simulink model "METI_Thermal_ver01_Jmaab_2018b"  (R2018b)
settings: Solver=ode8  StartTime=0  StopTime=end_time  FixedStep=sampling_time  RelTol=1e-3
PreLoadFcn:
  | %init_setting;
values from neighbouring files (symbols this model uses):
  degC2K = 273.15    [METI_TRAMI_Thermal_ver01_Jmaab_PreLoad.m]    (also in init_setting_METI.m)
  K2degC = -273.15    [METI_TRAMI_Thermal_ver01_Jmaab_PreLoad.m]    (also in init_setting_METI.m)
  sampling_time = 0.0025    [METI_TRAMI_Thermal_ver01_Jmaab_PreLoad.m]
undefined symbols (not defined in the file or in its folder): ACC_D_Gain, ACC_I_Gain, ACC_P_Gain, ALT_CNT_ALT_OFF_RPM_HYS_rpm, ALT_CNT_ALT_ON_RPM_HYS_rpm, ALT_CNT_Alter_V_BASE_V, ALT_CNT_Alter_V_Kaisei_V, ALT_CNT_flag_disable_kaisei, ALT_CNT_V_Battely_Kudo_V, ALT_PNT_ALT_GDCurrent_A, ALT_PNT_ALT_GDVolt_V, ALT_PNT_Alter_limit_Current_V_table, ALT_PNT_Alter_limit_Current_V_table_x_rpm, ALT_PNT_Alter_trq_Nm_map, ALT_PNT_Alter_trq_Nm_map_x_rpm, ALT_PNT_Alter_trq_Nm_map_y_Current_A, ALT_PNT_Alter_trq_Nm_map_z_Volt_tgt_V, ALT_PNT_eta_pulley_alt, ALT_PNT_Gain_Alt_v_del, ALT_PNT_ratio_pulley_alt, ALT_PNT_Tau_Alternator_V_tgt_s, ALT_PNT_trq_alter_output_LL_Nm, BK_PNT_Pow_UL, BK_PNT_Tau_brake, Brk_LL, Brk_PGain, Brk_UL, BT_PNT_Lo_Capa_lo_batt_F, BT_PNT_Lo_ocv_SOC_lo_batt_OCV_V_table, BT_PNT_Lo_ocv_SOC_lo_batt_OCV_V_table_x_SOC, BT_PNT_Lo_R_lo_batt_ohm, BT_PNT_Lo_SOC_MAX_lo_batt, BT_PNT_Lo_SOC_MIN_lo_batt, BT_PNT_Lo_SOC_START_lo_batt, BT_PNT_Lo_V_start_ocv, DF_PNT_DF_gear, DF_PNT_DFBlock2DFAir_Heat_Resi_KpW, DF_PNT_DFBlock_Heat_Capa_JpK, DF_PNT_DFBlock_Temp_ini_degC, DF_PNT_DFOil2DFBlock_Heat_Resi_KpW, DF_PNT_DFOil_Heat_Capa_JpK, DF_PNT_DFOil_Temp_ini_degC, DF_PNT_Driveshaft_damper, DF_PNT_Driveshaft_delta_radps_LL, DF_PNT_Driveshaft_delta_radps_UL, DF_PNT_Driveshaft_spring, DF_PNT_eta_DF, DF_PNT_Outtemp_degC, DF_PNT_TMBlock2DFBlock_Heat_Resi_KpW, Driver_Brake_Const1, Driver_Brake_Const3, Driver_Brake_Switch_Const2, Driver_Brk_sh, drivmode_ACC, drivmode_CONST, drivmode_GensokuKaisei, drivmode_GensokuRikko, drivmode_STOP, EL_PNT_R_bodyelec_lo_ohm, ENG_CNT_acc_idlestop ... (+137)
libraries: METI_Lib_vehicle_model x31, simulink x7, AZAPA_Lib_vehicle_model x1
(part 2 of 4)

== system METI_Thermal_ver01_Jmaab_2018b/Vehicle/CNT/ENG_CNT ==
  Driver_Input : Inport
  sensor_VL_PNT_BUS : Inport  Port=2
  sensor_ENG_PNT : Inport  Port=3
  Bus Creator : BusCreator  Inputs=4
  Bus Creator1 : BusCreator  Inputs=10
  Bus Selector1 : BusSelector  OutputSignals=flag_Lockup
  Bus Selector12 : BusSelector  OutputSignals=v_VL_PNT_kmph
  Bus Selector13 : BusSelector  OutputSignals=n_eng_rpm,fuel_consumption,T_ENGTH_PNT_Coolant_degC
  Bus Selector14 : BusSelector  OutputSignals=open_accel_per,open_brake_per
  ENG_Cntrl : Subsystem
  ENG_CNT_out : Outport
  tag scope: ENG_CNT_CAN_Tx=scoped
  wires:
  Bus Creator/1 -> [ENG_CNT_CAN_Tx]  "ENG_CNT_CAN_Tx"
  ENG_Cntrl/1(open_throttle_per) -> Bus Creator/1, Bus Creator1/1
  ENG_Cntrl/2(flag_IdleStop) -> Bus Creator/2, Bus Creator1/2
  ENG_Cntrl/3(flag_fuelcut) -> Bus Creator/3, Bus Creator1/3
  ENG_Cntrl/4(fuel_ratio) -> Bus Creator1/4
  ENG_Cntrl/5(timing_ignition) -> Bus Creator1/5
  ENG_Cntrl/6(n_eng_rpm) -> Bus Creator/4, Bus Creator1/6
  ENG_Cntrl/7(flag_ON_Starter) -> Bus Creator1/7
  Bus Creator1/1 -> ENG_CNT_out/1  "ENG_CNT_out"
  sensor_ENG_PNT/1 -> Bus Selector13/1
  Bus Selector13/1 -> ENG_Cntrl/3(sens_ENG_PNT)  "<n_eng_rpm>"
  sensor_VL_PNT_BUS/1 -> Bus Selector12/1
  Bus Selector12/1 -> ENG_Cntrl/6(v_VL_PNT_kmph)  "<v_VL_PNT_kmph>"
  Driver_Input/1 -> Bus Selector14/1
  Bus Selector14/1 -> ENG_Cntrl/1(open_accel_per)  "<open_accel_per>"
  Bus Selector14/2 -> ENG_Cntrl/2(open_brake_per)  "<open_brake_per>"
  [ENG_CNT_CAN_Rx] -> Bus Selector1/1
  Bus Selector1/1 -> ENG_Cntrl/7(flag_Lockup)  "<flag_Lockup>"
  ENG_Cntrl/8(K_Fuel) -> Bus Creator1/8
  ENG_Cntrl/9(V_ENG_CNT_WP_V) -> Bus Creator1/9
  ENG_Cntrl/10(V_ENG_CNT_RDFan_V) -> Bus Creator1/10
  Bus Selector13/2 -> ENG_Cntrl/4(fuel_consumption)  "<fuel_consumption>"
  Bus Selector13/3 -> ENG_Cntrl/5(T_ENGTH_PNT_Coolant_K)  "<T_ENGTH_PNT_Coolant_degC>"

== system METI_Thermal_ver01_Jmaab_2018b/Vehicle/CNT/TM_CNT ==
  sensor_VL_PNT_BUS : Inport
  sensor_ENG_PNT : Inport  Port=2
  sensor_TM_PNT_BUS : Inport  Port=3
  Bus Creator : BusCreator  Inputs=2
  Bus Creator1 : BusCreator  Inputs=4
  Bus Selector1 : BusSelector  OutputSignals=open_throttle_per
  Bus Selector2 : BusSelector  OutputSignals=n_TM_PNT_rpm,T_TMTH_PNT_CVTF_degC
  Bus Selector3 : BusSelector  OutputSignals=v_VL_PNT_kmph
  Bus Selector4 : BusSelector  OutputSignals=T_ENGTH_PNT_Coolant_degC
  TM_Ctrl : Subsystem
  TM_CNT_out : Outport
  tag scope: TM_CNT_CAN_Tx=scoped
  wires:
  Bus Creator/1 -> [TM_CNT_CAN_Tx]  "TM_CNT_CAN_Tx"
  [TM_CNT_CAN_Rx] -> Bus Selector1/1
  Bus Selector1/1 -> TM_Ctrl/5(open_throttle_per)  "<open_throttle_per>"
  TM_Ctrl/1(flag_Lockup) -> Bus Creator1/1, Bus Creator/1
  TM_Ctrl/2(omg_Slip_rpm) -> Bus Creator1/2, Bus Creator/2
  TM_Ctrl/3(ratio_CVT) -> Bus Creator1/3
  Bus Creator1/1 -> TM_CNT_out/1  "TM_CNT_out"
  sensor_VL_PNT_BUS/1 -> Bus Selector3/1
  Bus Selector3/1 -> TM_Ctrl/1(v_VL_PNT_kmph)  "<v_VL_PNT_kmph>"
  sensor_TM_PNT_BUS/1 -> Bus Selector2/1
  Bus Selector2/1 -> TM_Ctrl/2(n_TM_PNT_rpm)  "<n_TM_PNT_rpm>"
  TM_Ctrl/4(R_CVTF_warmer_tgt_KpW) -> Bus Creator1/4
  sensor_ENG_PNT/1 -> Bus Selector4/1
  Bus Selector2/2 -> TM_Ctrl/3(T_TMTH_PNT_CVTF_K)  "<T_TMTH_PNT_CVTF_degC>"
  Bus Selector4/1 -> TM_Ctrl/4(T_ENG_Coolant_K)  "<T_ENGTH_PNT_Coolant_degC>"

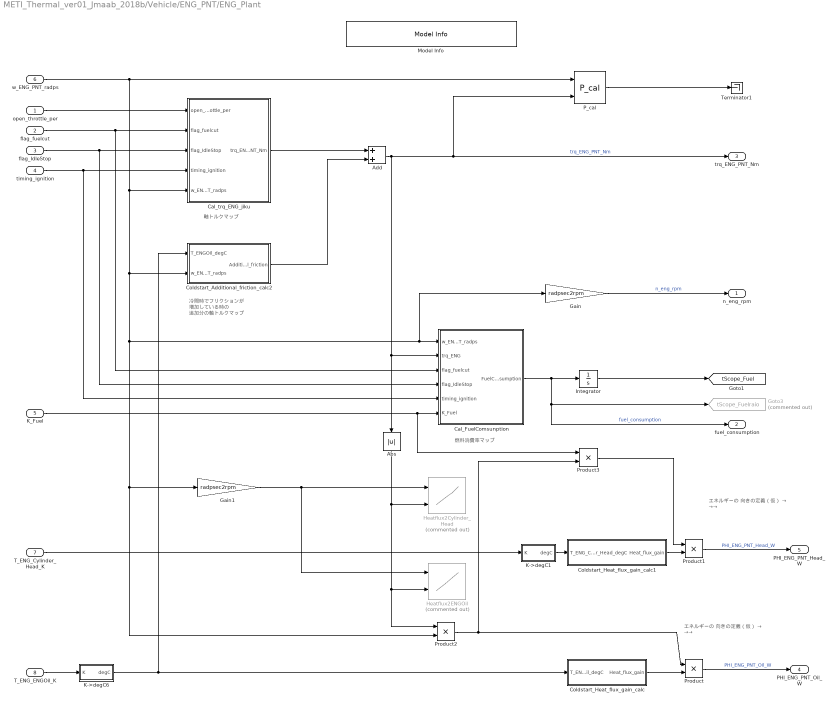
== system METI_Thermal_ver01_Jmaab_2018b/Vehicle/ENG_PNT/ENG_Plant ==
  note: 軸トルクマップ
  note: 燃料消費率マップ
  note: 冷間時でフリクションが
      | 増加している時の
      | 追加分の軸トルクマップ
  note: エネルギーの
      | 向きの定義（仮）
      | → →→
  note: エネルギーの
      | 向きの定義（仮）
      | → →→
  open_throttle_per : Inport
  flag_fuelcut : Inport  Port=2
  flag_IdleStop : Inport  Port=3
  timing_ignition : Inport  Port=4
  K_Fuel : Inport  Port=5
  w_ENG_PNT_radps : Inport  Port=6
  T_ENG_Cylinder_Head_K : Inport  Port=7
  T_ENG_ENGOil_K : Inport  Port=8
  Abs : Abs
  Add : Sum
  Cal_FuelComsunption : Subsystem
  Cal_trq_ENG_jiku : Subsystem
  Coldstart_Additional_friction_calc2 : Subsystem
  Coldstart_Heat_flux_gain_calc : Subsystem
  Coldstart_Heat_flux_gain_calc1 : Subsystem
  Gain : Gain  Gain=radpsec2rpm
  Gain1 : Gain  Gain=radpsec2rpm
  Goto3 : Goto  Commented=on  GotoTag=tScope_Fuelraio  TagVisibility=global
  Heatflux2Cylinder_Head : Lookup_n-D  Commented=on  BreakpointsForDimension1=ENG_PNT_Heatflux2Cylinder_Head_W_x_rpm  BreakpointsForDimension2=ENG_PNT_Heatflux2Cylinder_Head_W_y_trq  Table=ENG_PNT_Heatflux2Cylinder_Head_W  InternalRulePriority=Speed  RndMeth=Simplest  InputSameDT=on
  Heatflux2ENGOil : Lookup_n-D  Commented=on  BreakpointsForDimension1=ENG_PNT_Heatflux2ENGOil_W_x_rpm  BreakpointsForDimension2=ENG_PNT_Heatflux2ENGOil_W_y_trq  Table=ENG_PNT_Heatflux2ENGOil_W  InternalRulePriority=Speed  RndMeth=Simplest  InputSameDT=on
  Integrator : Integrator
  K->degC1 : Subsystem
  K->degC6 : Subsystem
  Model Info : simulink/Model-Wide Utilities/Model Info  Frame=on  DisplayStringWithTags=【注記】 ・エンジンモデルはトルク出力動作させる側が正  HorizontalTextAlignment=Left  LeftAlignmentValue=0.02
  P_cal : METI_Lib_vehicle_model/P_cal  Type_energy=回転運動  Type_output_energy=出力  Power_name=Po_  t_Workspace_Name=ENG_PNT_MECK  P_VariableName=Po_ENG_PNT_MECK  Across_VariableName=w_ENG_PNT_MECK  Throgh_VariableName=tq_ENG_PNT_MECK
  Product{,1..3} (4 alike) : Product
  Terminator1 : Terminator
  n_eng_rpm : Outport
  fuel_consumption : Outport  Port=2
  trq_ENG_PNT_Nm : Outport  Port=3
  PHI_ENG_PNT_Oil_W : Outport  Port=4
  PHI_ENG_PNT_Head_W : Outport  Port=5
  tag scope: tScope_Fuel=global
  wires:
  Cal_FuelComsunption/1(FuelConsumption) -> fuel_consumption/1, Goto3/1, Integrator/1  "fuel_consumption"
  Integrator/1 -> [tScope_Fuel]
  w_ENG_PNT_radps/1 -> P_cal/1, Coldstart_Additional_friction_calc2/2(w_ENG_PNT_radps), Gain1/1, Product2/2, Gain/1, Cal_FuelComsunption/1(w_ENG_PNT_radps), Cal_trq_ENG_jiku/5(w_ENG_PNT_radps)
  P_cal/1 -> Terminator1/1
  flag_fuelcut/1 -> Cal_trq_ENG_jiku/2(flag_fuelcut), Cal_FuelComsunption/3(flag_fuelcut)
  flag_IdleStop/1 -> Cal_FuelComsunption/4(flag_IdleStop), Cal_trq_ENG_jiku/3(flag_IdleStop)
  open_throttle_per/1 -> Cal_trq_ENG_jiku/1(open_throttle_per)
  Cal_trq_ENG_jiku/1(trq_ENG_PNT_Nm) -> Add/1
  timing_ignition/1 -> Cal_FuelComsunption/5(timing_ignition), Cal_trq_ENG_jiku/4(timing_ignition)
  Gain/1 -> n_eng_rpm/1  "n_eng_rpm"
  K->degC6/1(degC) -> Coldstart_Heat_flux_gain_calc/1(T_ENGOil_degC), Coldstart_Additional_friction_calc2/1(T_ENGOil_degC)
  T_ENG_Cylinder_Head_K/1 -> K->degC1/1(K)
  Product1/1 -> PHI_ENG_PNT_Head_W/1  "PHI_ENG_PNT_Head_W"
  Product/1 -> PHI_ENG_PNT_Oil_W/1  "PHI_ENG_PNT_Oil_W"
  Gain1/1 -> Heatflux2ENGOil/1, Heatflux2Cylinder_Head/1
  Coldstart_Heat_flux_gain_calc/1(Heat_flux_gain) -> Product/2
  Product2/1 -> Product/1, Product3/2
  Coldstart_Heat_flux_gain_calc1/1(Heat_flux_gain) -> Product1/2
  Coldstart_Additional_friction_calc2/1(Additional_friction) -> Add/2
  Add/1 -> trq_ENG_PNT_Nm/1, P_cal/2, Cal_FuelComsunption/2(trq_ENG), Abs/1  "trq_ENG_PNT_Nm"
  K_Fuel/1 -> Product3/1, Cal_FuelComsunption/6(K_Fuel)
  Abs/1 -> Product2/1, Heatflux2ENGOil/2, Heatflux2Cylinder_Head/2
  Product3/1 -> Product1/1
  T_ENG_ENGOil_K/1 -> K->degC6/1(K)
  K->degC1/1(degC) -> Coldstart_Heat_flux_gain_calc1/1(T_ENG_Cylinder_Head_degC)

== system METI_Thermal_ver01_Jmaab_2018b/Vehicle/ENG_PNT/K->degC ==
  K : Inport
  Constant2 : Constant  Value=K2degC
  Sum : Sum  Inputs=++|
  degC : Outport
  wires:
  K/1 -> Sum/2
  Constant2/1 -> Sum/1
  Sum/1 -> degC/1

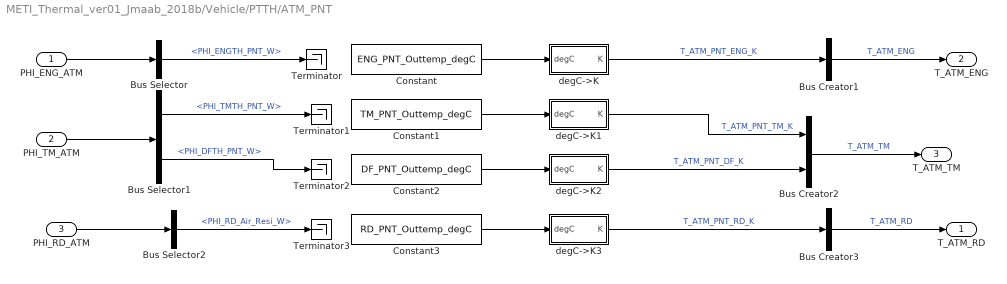
== system METI_Thermal_ver01_Jmaab_2018b/Vehicle/PTTH/ATM_PNT ==
  PHI_ENG_ATM : Inport
  PHI_TM_ATM : Inport  Port=2
  PHI_RD_ATM : Inport  Port=3
  Bus Creator1 : BusCreator  Inputs=1
  Bus Creator2 : BusCreator  Inputs=2
  Bus Creator3 : BusCreator  Inputs=1
  Bus Selector : BusSelector  OutputSignals=PHI_ENGTH_PNT_W
  Bus Selector1 : BusSelector  OutputSignals=PHI_TMTH_PNT_W,PHI_DFTH_PNT_W
  Bus Selector2 : BusSelector  OutputSignals=PHI_RD_Air_Resi_W
  Constant : Constant  Value=ENG_PNT_Outtemp_degC
  Constant1 : Constant  Value=TM_PNT_Outtemp_degC
  Constant2 : Constant  Value=DF_PNT_Outtemp_degC
  Constant3 : Constant  Value=RD_PNT_Outtemp_degC
  Terminator{,1..3} (4 alike) : Terminator
  degC->K : Subsystem
  degC->K1 : Subsystem
  degC->K2 : Subsystem
  degC->K3 : Subsystem
  T_ATM_RD : Outport
  T_ATM_ENG : Outport  Port=2
  T_ATM_TM : Outport  Port=3
  wires:
  Constant/1 -> degC->K/1(degC)
  Constant1/1 -> degC->K1/1(degC)
  Constant2/1 -> degC->K2/1(degC)
  Constant3/1 -> degC->K3/1(degC)
  Bus Selector1/2 -> Terminator2/1  "<PHI_DFTH_PNT_W>"
  degC->K/1(K) -> Bus Creator1/1  "T_ATM_PNT_ENG_K"
  degC->K1/1(K) -> Bus Creator2/1  "T_ATM_PNT_TM_K"
  degC->K2/1(K) -> Bus Creator2/2  "T_ATM_PNT_DF_K"
  degC->K3/1(K) -> Bus Creator3/1  "T_ATM_PNT_RD_K"
  PHI_ENG_ATM/1 -> Bus Selector/1
  Bus Selector/1 -> Terminator/1  "<PHI_ENGTH_PNT_W>"
  PHI_TM_ATM/1 -> Bus Selector1/1
  Bus Selector1/1 -> Terminator1/1  "<PHI_TMTH_PNT_W>"
  Bus Creator2/1 -> T_ATM_TM/1  "T_ATM_TM"
  Bus Creator1/1 -> T_ATM_ENG/1  "T_ATM_ENG"
  Bus Creator3/1 -> T_ATM_RD/1  "T_ATM_RD"
  PHI_RD_ATM/1 -> Bus Selector2/1
  Bus Selector2/1 -> Terminator3/1  "<PHI_RD_Air_Resi_W>"

== system METI_Thermal_ver01_Jmaab_2018b/Vehicle/PTTH/DTTH_PNT ==
  note: DFブロックへ
      | 放熱する熱量
  note: CVTFからエンジン冷却水へ
      | 放熱する熱量
  note: エンジンブロックからT/Mブロックへ
      | 放熱する熱量
  note: エネルギーの
      | 向きの定義（仮）
      | →→→
  note: エネルギーの
      | 向きの定義（仮）
      | →→→
  note: エネルギーの
      | 向きの定義（仮）
      | →→→
  note: T/MからCVTFへ
      | 放熱する熱量
  note: DFの損失が
      | DFオイルへの熱量
  TM_CNT_out : Inport
  T_ATM_TM : Inport  Port=2
  T_ENG_TM : Inport  Port=3
  PHI_TM_PNT_BUS : Inport  Port=4
  Bus Creator{1..4} (4 alike) : BusCreator  Inputs=2
  Bus Selector1 : BusSelector  OutputSignals=T_ENG_Block_K,T_ENGTH_PNT_Coolant_K
  Bus Selector2 : BusSelector  OutputSignals=R_CVTF_warmer_tgt_KpW
  Bus Selector3 : BusSelector  OutputSignals=Q_Tire_rol_resi,W_TM_PNT_W
  Bus Selector4 : BusSelector  OutputSignals=T_ATM_PNT_TM_K,T_ATM_PNT_DF_K
  DFTH_PNT : Subsystem
      mask Display: image(imread('picture\differential.png'))
  TMTH_PNT : Subsystem
      mask Display: image(imread('picture\image\transmission02.jpg'))
  Terminator : Terminator
  T_TMTH_PNT : Outport
  PHI_TM_ATM : Outport  Port=2
  PHI_TM_ENG : Outport  Port=3
  TMTH_Info : Outport  Port=4
  wires:
  DFTH_PNT/2(PHI_DFTH_PNT_W) -> Bus Creator3/1
  Bus Selector4/2 -> DFTH_PNT/3(T_ATM_PNT_DF_K)  "<T_ATM_PNT_DF_K>"
  TMTH_PNT/4(T_TMTH_PNT_CVTF_K) -> Terminator/1
  TMTH_PNT/2(T_TM_Block0_K) -> DFTH_PNT/1(T_DF_Block_K)
  DFTH_PNT/1(PHI_DF_Block_W) -> TMTH_PNT/1(W_TM_Block0_W)
  TMTH_PNT/6(PHI_TMTH_PNT_W) -> Bus Creator3/2
  TMTH_PNT/5(PHI_ENGBlock_Resi2_W) -> Bus Creator1/2
  TMTH_PNT/3(PHI_TM_CVTF_Resi_W) -> Bus Creator1/1
  T_ENG_TM/1 -> Bus Selector1/1
  Bus Selector1/1 -> TMTH_PNT/4(T_TM_Block_Resi_K)  "<T_ENG_Block_K>"
  Bus Selector1/2 -> TMTH_PNT/5(T_ENGTH_PNT_Coolant_K)  "<T_ENGTH_PNT_Coolant_K>"
  TMTH_PNT/1(T_TMTH_PNT_CVTF1_K) -> Bus Creator4/1, Bus Creator2/1  "T_TMTH_PNT_CVTF_K"
  DFTH_PNT/3(T_DFBlock_K) -> Bus Creator4/2, Bus Creator2/2  "T_DFBlock_K"
  Bus Creator2/1 -> T_TMTH_PNT/1  "T_TMTH_PNT"
  Bus Creator1/1 -> PHI_TM_ENG/1  "PHI_TM_ENG"
  Bus Creator3/1 -> PHI_TM_ATM/1  "PHI_TM_ATM"
  Bus Creator4/1 -> TMTH_Info/1  "TMTH_Info"
  PHI_TM_PNT_BUS/1 -> Bus Selector3/1
  Bus Selector3/2 -> TMTH_PNT/3(PHI_TM_PNT_W)  "<W_TM_PNT_W>"
  Bus Selector3/1 -> DFTH_PNT/2(PHI_DF_PNT_W)  "<Q_Tire_rol_resi>"
  TM_CNT_out/1 -> Bus Selector2/1
  Bus Selector2/1 -> TMTH_PNT/2(R_CVTF_warmer_tgt_KpW)  "<R_CVTF_warmer_tgt_KpW>"
  T_ATM_TM/1 -> Bus Selector4/1
  Bus Selector4/1 -> TMTH_PNT/6(T_ATM_PNT_TM_K)  "<T_ATM_PNT_TM_K>"

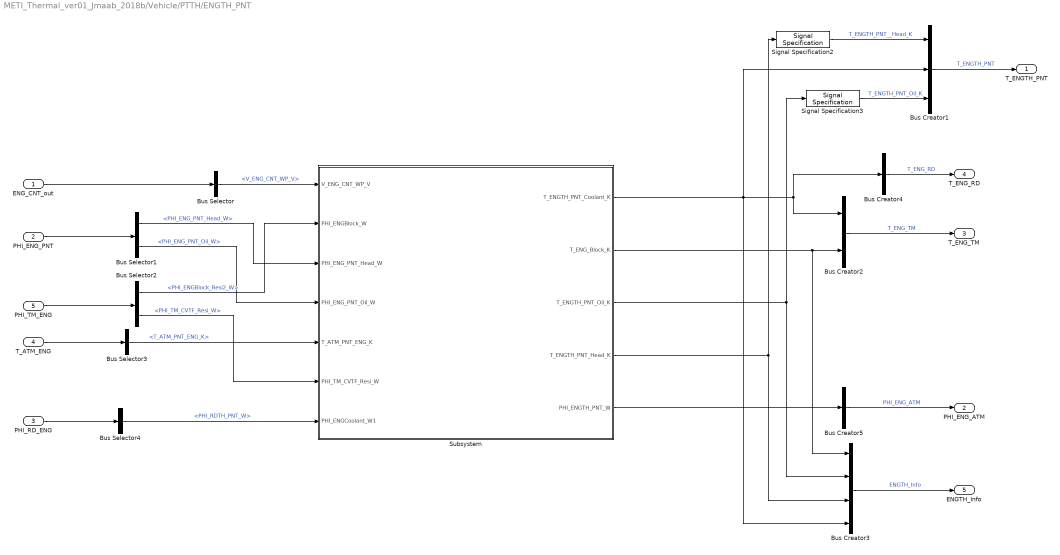
== system METI_Thermal_ver01_Jmaab_2018b/Vehicle/PTTH/ENGTH_PNT ==
  ENG_CNT_out : Inport
  PHI_ENG_PNT : Inport  Port=2
  PHI_RD_ENG : Inport  Port=3
  T_ATM_ENG : Inport  Port=4
  PHI_TM_ENG : Inport  Port=5
  Bus Creator1 : BusCreator  Inputs=3
  Bus Creator2 : BusCreator  Inputs=2
  Bus Creator3 : BusCreator  Inputs=4
  Bus Creator4 : BusCreator  Inputs=1
  Bus Creator5 : BusCreator  Inputs=1
  Bus Selector : BusSelector  OutputSignals=V_ENG_CNT_WP_V
  Bus Selector1 : BusSelector  OutputSignals=PHI_ENG_PNT_Head_W,PHI_ENG_PNT_Oil_W
  Bus Selector2 : BusSelector  OutputSignals=PHI_ENGBlock_Resi2_W,PHI_TM_CVTF_Resi_W
  Bus Selector3 : BusSelector  OutputSignals=T_ATM_PNT_ENG_K
  Bus Selector4 : BusSelector  OutputSignals=PHI_RDTH_PNT_W
  Signal Specification2 : SignalSpecification
  Signal Specification3 : SignalSpecification
  Subsystem : Subsystem
  T_ENGTH_PNT : Outport
  PHI_ENG_ATM : Outport  Port=2
  T_ENG_TM : Outport  Port=3
  T_ENG_RD : Outport  Port=4
  ENGTH_Info : Outport  Port=5
  wires:
  ENG_CNT_out/1 -> Bus Selector/1
  Subsystem/1(T_ENGTH_PNT_Coolant_K) -> Bus Creator3/4, Bus Creator1/2, Bus Creator2/1, Bus Creator4/1
  Subsystem/2(T_ENG_Block_K) -> Bus Creator3/1, Bus Creator2/2
  Subsystem/3(T_ENGTH_PNT_Oil_K) -> Bus Creator3/2, Signal Specification3/1
  Subsystem/4(T_ENGTH_PNT_Head_K) -> Bus Creator3/3, Signal Specification2/1
  Subsystem/5(PHI_ENGTH_PNT_W) -> Bus Creator5/1
  Bus Selector/1 -> Subsystem/1(V_ENG_CNT_WP_V)  "<V_ENG_CNT_WP_V>"
  PHI_ENG_PNT/1 -> Bus Selector1/1
  Bus Selector1/1 -> Subsystem/3(PHI_ENG_PNT_Head_W)  "<PHI_ENG_PNT_Head_W>"
  Bus Selector1/2 -> Subsystem/4(PHI_ENG_PNT_Oil_W)  "<PHI_ENG_PNT_Oil_W>"
  Bus Creator1/1 -> T_ENGTH_PNT/1  "T_ENGTH_PNT"
  Signal Specification2/1 -> Bus Creator1/1  "T_ENGTH_PNT__Head_K"
  Signal Specification3/1 -> Bus Creator1/3  "T_ENGTH_PNT_Oil_K"
  Bus Creator2/1 -> T_ENG_TM/1  "T_ENG_TM"
  Bus Creator4/1 -> T_ENG_RD/1  "T_ENG_RD"
  Bus Creator5/1 -> PHI_ENG_ATM/1  "PHI_ENG_ATM"
  Bus Creator3/1 -> ENGTH_Info/1  "ENGTH_Info"
  PHI_TM_ENG/1 -> Bus Selector2/1
  Bus Selector2/1 -> Subsystem/2(PHI_ENGBlock_W)  "<PHI_ENGBlock_Resi2_W>"
  Bus Selector2/2 -> Subsystem/6(PHI_TM_CVTF_Resi_W)  "<PHI_TM_CVTF_Resi_W>"
  T_ATM_ENG/1 -> Bus Selector3/1
  PHI_RD_ENG/1 -> Bus Selector4/1
  Bus Selector3/1 -> Subsystem/5(T_ATM_PNT_ENG_K)  "<T_ATM_PNT_ENG_K>"
  Bus Selector4/1 -> Subsystem/7(PHI_ENGCoolant_W1)  "<PHI_RDTH_PNT_W>"

== system METI_Thermal_ver01_Jmaab_2018b/Vehicle/PTTH/RDTH_PNT ==
  ENG_CNT_out : Inport
  T_ENG_RD : Inport  Port=2
  v_VL_PNT_kmph : Inport  Port=3
  T_ATM_RD : Inport  Port=4
  Bus Creator1 : BusCreator  Inputs=1
  Bus Creator2 : BusCreator  Inputs=1
  Bus Creator4 : BusCreator  Inputs=2
  Bus Selector : BusSelector  OutputSignals=V_ENG_CNT_RDFan_V
  Bus Selector1 : BusSelector  OutputSignals=T_ENGTH_PNT_Coolant_K
  Bus Selector2 : BusSelector  OutputSignals=T_ATM_PNT_RD_K
  Subsystem : Subsystem
  mps2kmph : Gain  Gain=mps2kmph
  PHI_RD_ENG : Outport
  PHI_RD_ATM : Outport  Port=2
  RDTH_Info : Outport  Port=3
  wires:
  v_VL_PNT_kmph/1 -> mps2kmph/1
  Subsystem/1(T_RDCoolant_degC) -> Bus Creator4/1
  Subsystem/2(PHI_RDTH_PNT_W) -> Bus Creator4/2, Bus Creator1/1
  Subsystem/3(PHI_RD_Air_Resi_W) -> Bus Creator2/1
  ENG_CNT_out/1 -> Bus Selector/1
  Bus Selector/1 -> Subsystem/1(RD_PNT_Voltage_RDFan_V)  "<V_ENG_CNT_RDFan_V>"
  T_ENG_RD/1 -> Bus Selector1/1
  Bus Selector1/1 -> Subsystem/3(T_ENGTH_PNT_Coolant_K)  "<T_ENGTH_PNT_Coolant_K>"
  mps2kmph/1 -> Subsystem/2(v_VL_PNT_kmph)  "v_VL_PNT_kmph"
  Bus Creator4/1 -> RDTH_Info/1  "RDTH_Info"
  Bus Creator1/1 -> PHI_RD_ENG/1  "PHI_RD_ENG"
  Bus Creator2/1 -> PHI_RD_ATM/1  "PHI_RD_ATM"
  T_ATM_RD/1 -> Bus Selector2/1
  Bus Selector2/1 -> Subsystem/4(T_ATM_PNT_RD_K)  "<T_ATM_PNT_RD_K>"

== system METI_Thermal_ver01_Jmaab_2018b/Vehicle/TM_PNT/DF_PNT ==
  note: DF効率
  note: 車両を動かす側が正
  w_DF_PNT_DN_radps : Inport
  w_DF_PNT_UP_radps : Inport  Port=2
  T_DF_PNT_K : Inport  Port=3
  Constant4 : Constant  Value=DF_PNT_DF_gear
  DriveShaft : Subsystem
  Product4 : Product  Inputs=*/  RndMeth=Zero
  Product7 : Product  Inputs=*/  RndMeth=Zero
  Q_cal1 : METI_Lib_vehicle_model/P_cal  Type_energy=回転運動  Type_output_energy=出力  Power_name=Po_  t_Workspace_Name=DF_PNT_MECK  P_VariableName=Po_DF_PNT_MECK  Across_VariableName=w_DF_PNT_MECK  Throgh_VariableName=tq_DF_PNT_MECK
  Q_cal4 : METI_Lib_vehicle_model/P_cal  Type_energy=回転運動  Type_output_energy=損失  Power_name=Pl_  t_Workspace_Name=DF_PNT_MECK_LOSS  P_VariableName=Pl_DF_PNT_MECK_LOSS  Across_VariableName=w_DF_PNT_MECK_LOSS  Throgh_VariableName=tq_DF_PNT_MECK_LOSS
  Terminator : Terminator
  Terminator3 : Terminator
  eta_DF : Constant  Value=DF_PNT_eta_DF
  eta_cal : METI_Lib_vehicle_model/eta_cal  SystemSampleTime=-1
  trq_DS_PNT_Nm : Outport
  trq_DFNT_Nm : Outport  Port=2
  PHI_DF_PNT_W : Outport  Port=3
  wires:
  w_DF_PNT_UP_radps/1 -> Product4/1, Q_cal4/1, Q_cal1/1
  eta_DF/1 -> eta_cal/1
  eta_cal/2 -> Q_cal1/2, trq_DFNT_Nm/1  "trq_DFNT_Nm"
  eta_cal/1 -> Q_cal4/2
  Q_cal1/1 -> Terminator3/1
  Constant4/1 -> Product7/2, Product4/2
  Product7/1 -> eta_cal/2
  DriveShaft/1(trq_DS_PNT_in_Nm) -> trq_DS_PNT_Nm/1  "trq_DS_PNT_Nm"
  Product4/1 -> DriveShaft/2(w_DS_PNT_in_radps)
  w_DF_PNT_DN_radps/1 -> DriveShaft/1(w_TR_PNT_radps)
  DriveShaft/2(trq_DF_PNT_Nm) -> Product7/1
  Q_cal4/1 -> PHI_DF_PNT_W/1
  T_DF_PNT_K/1 -> Terminator/1

== system METI_Thermal_ver01_Jmaab_2018b/Vehicle/TM_PNT/K->degC ==
  K : Inport
  Constant2 : Constant  Value=K2degC
  Sum : Sum  Inputs=++|
  degC : Outport
  wires:
  K/1 -> Sum/2
  Constant2/1 -> Sum/1
  Sum/1 -> degC/1

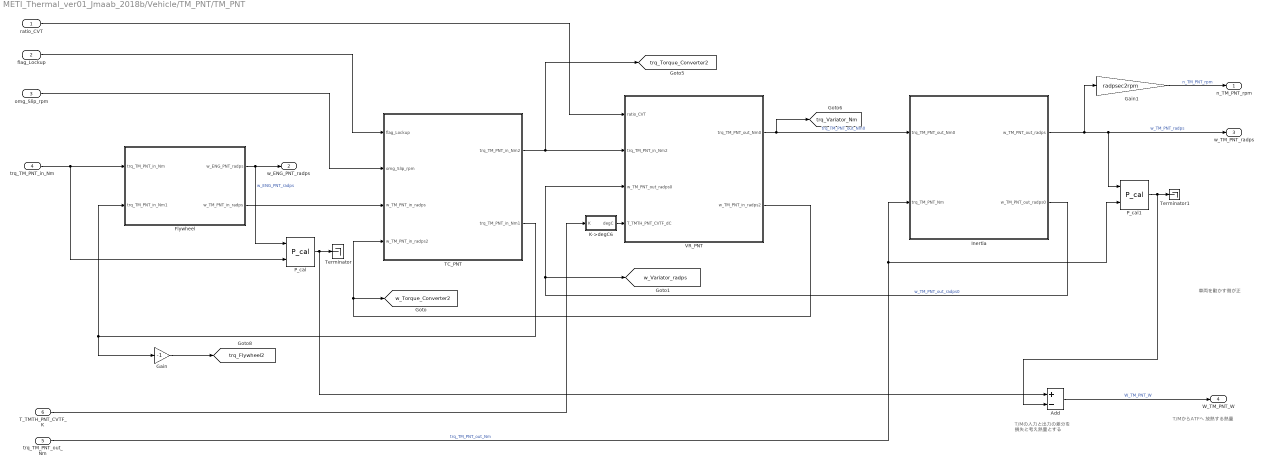
== system METI_Thermal_ver01_Jmaab_2018b/Vehicle/TM_PNT/TM_PNT ==
  note: 車両を動かす側が正
  note: T/MからATFへ
      | 放熱する熱量
  note: T/Mの入力と出力の差分を
      | 損失と考え熱量とする
  ratio_CVT : Inport
  flag_Lockup : Inport  Port=2
  omg_Slip_rpm : Inport  Port=3
  trq_TM_PNT_in_Nm : Inport  Port=4
  trq_TM_PNT_out_Nm : Inport  Port=5
  T_TMTH_PNT_CVTF_K : Inport  Port=6
  Add : Sum  Inputs=+-
  Flywheel : Subsystem
  Gain : Gain  Gain=-1
  Gain1 : Gain  Gain=radpsec2rpm
  Inertia : Subsystem
  K->degC6 : Subsystem
  P_cal : METI_Lib_vehicle_model/P_cal  Type_energy=回転運動  Type_output_energy=出力  Power_name=Po_  t_Workspace_Name=TM_PNT_MECK_UP  P_VariableName=Po_TM_PNT_MECK_UP  Across_VariableName=w_TM_PNT_MECK_UP  Throgh_VariableName=tq_TM_PNT_MECK_UP
  P_cal1 : METI_Lib_vehicle_model/P_cal  Type_energy=回転運動  Type_output_energy=出力  Power_name=Po_  t_Workspace_Name=TM_PNT_MECK_DN  P_VariableName=Po_TM_PNT_MECK_DN  Across_VariableName=w_TM_PNT_MECK_DN  Throgh_VariableName=tq_TM_PNT_MECK_DN
  TC_PNT : Subsystem
  Terminator : Terminator
  Terminator1 : Terminator
  VR_PNT : Subsystem
  n_TM_PNT_rpm : Outport
  w_ENG_PNT_radps : Outport  Port=2
  w_TM_PNT_radps : Outport  Port=3
  W_TM_PNT_W : Outport  Port=4
  tag scope: trq_Flywheel2=global, trq_Torque_Converter2=global, trq_Variator_Nm=global, w_Torque_Converter2=global, w_Variator_radps=global
  wires:
  VR_PNT/2(w_TM_PNT_in_radps2) -> [w_Torque_Converter2], TC_PNT/4(w_TM_PNT_in_radps2)
  TC_PNT/1(trq_TM_PNT_in_Nm2) -> [trq_Torque_Converter2], VR_PNT/2(trq_TM_PNT_in_Nm2)
  flag_Lockup/1 -> TC_PNT/1(flag_Lockup)
  omg_Slip_rpm/1 -> TC_PNT/2(omg_Slip_rpm)
  ratio_CVT/1 -> VR_PNT/1(ratio_CVT)
  TC_PNT/2(trq_TM_PNT_in_Nm1) -> Gain/1, Flywheel/2(trq_TM_PNT_in_Nm1)
  Flywheel/2(w_TM_PNT_in_radps) -> TC_PNT/3(w_TM_PNT_in_radps)
  Flywheel/1(w_ENG_PNT_radps) -> w_ENG_PNT_radps/1, P_cal/1  "w_ENG_PNT_radps"
  trq_TM_PNT_in_Nm/1 -> P_cal/2, Flywheel/1(trq_TM_PNT_in_Nm)
  Inertia/1(w_TM_PNT_out_radps) -> w_TM_PNT_radps/1, P_cal1/1, Gain1/1  "w_TM_PNT_radps"
  Gain1/1 -> n_TM_PNT_rpm/1  "n_TM_PNT_rpm"
  P_cal/1 -> Add/1, Terminator/1
  P_cal1/1 -> Terminator1/1, Add/2
  trq_TM_PNT_out_Nm/1 -> Inertia/2(trq_TM_PNT_Nm), P_cal1/2  "trq_TM_PNT_out_Nm"
  Inertia/2(w_TM_PNT_out_radps0) -> [w_Variator_radps], VR_PNT/3(w_TM_PNT_out_radps0)  "w_TM_PNT_out_radps0"
  VR_PNT/1(trq_TM_PNT_out_Nm0) -> [trq_Variator_Nm], Inertia/1(trq_TM_PNT_out_Nm0)  "trq_TM_PNT_out_Nm0"
  Add/1 -> W_TM_PNT_W/1  "W_TM_PNT_W"
  T_TMTH_PNT_CVTF_K/1 -> K->degC6/1(K)
  Gain/1 -> [trq_Flywheel2]
  K->degC6/1(degC) -> VR_PNT/4(T_TMTH_PNT_CVTF_dC)

== system METI_Thermal_ver01_Jmaab_2018b/Driver/Caliculate_Opeining_Accel/FB/Filter ==
  In1 : Inport
  Gain3 : Gain  Gain=10
  Gain4 : Gain  Gain=0.1
  Rounding Function : Rounding  Operator=round
  Out1 : Outport
  wires:
  Rounding Function/1 -> Gain4/1
  In1/1 -> Gain3/1
  Gain3/1 -> Rounding Function/1
  Gain4/1 -> Out1/1

== system METI_Thermal_ver01_Jmaab_2018b/Driver/Caliculate_Opeining_Accel/FF/Air_Resistance ==
  V_tgt : Inport
  V_wind : Constant  Value=VL_PNT_V_wind
  cal_Air_resi1 : METI_Lib_vehicle_model/vehicle_model/cal_Air_resi  Vel_max=200
  F_air_resi : Outport
  wires:
  V_tgt/1 -> cal_Air_resi1/1
  V_wind/1 -> cal_Air_resi1/2
  cal_Air_resi1/1 -> F_air_resi/1

== system METI_Thermal_ver01_Jmaab_2018b/Driver/Caliculate_Opeining_Accel/FF/Cal_M_ENG_jiku2 ==
  note: 軸トルクマップ
  FF_trq_accel_Nm : Inport
  pre_n_eng_rpm : Inport  Port=2
  2-D Lookup Table : Lookup_n-D  BreakpointsForDimension1=ENG_trq_rev  BreakpointsForDimension2=ENG_rpm  Table=ENG_throttle_rev  ExtrapMethod=Clip  UseLastTableValue=on  RndMeth=Simplest  InputSameDT=on
  2-D Lookup Table1 : Lookup_n-D  BreakpointsForDimension1=ENG_PNT_trq_Nm_map_y_throttle  BreakpointsForDimension2=ENG_PNT_trq_Nm_map_x_rpm  Table=ENG_PNT_trq_Nm_map  ExtrapMethod=Clip  UseLastTableValue=on  RndMeth=Simplest  InputSameDT=on
  Constant : Constant  Value=0
  Subsystem : Subsystem
  Sum : Sum  Inputs=|++
  FF_open_accel_per : Outport
  wires:
  FF_trq_accel_Nm/1 -> Sum/1
  2-D Lookup Table/1 -> Subsystem/1(In1)
  pre_n_eng_rpm/1 -> 2-D Lookup Table/2, 2-D Lookup Table1/2
  Constant/1 -> 2-D Lookup Table1/1
  Sum/1 -> 2-D Lookup Table/1
  2-D Lookup Table1/1 -> Sum/2
  Subsystem/1(Out1) -> FF_open_accel_per/1

== system METI_Thermal_ver01_Jmaab_2018b/Driver/Caliculate_Opeining_Accel/FF/Inertial_Resistance ==
  V_tgt : Inport
  Constant : Constant  Value=M
  Derivative : Derivative
  Divide : Product  OutDataTypeStr=Inherit: Same as first input
  F_Inertia : Outport
  wires:
  Constant/1 -> Divide/2
  Derivative/1 -> Divide/1
  Divide/1 -> F_Inertia/1
  V_tgt/1 -> Derivative/1

== system METI_Thermal_ver01_Jmaab_2018b/Driver/Caliculate_Opeining_Accel/FF/Rolling_Resistance ==
  note: 20151211修正
      |
      | 空気抵抗と表現を統一する、ため
      | -1のGainを削除
  V_tgt : Inport
  cal_roll_resi1 : METI_Lib_vehicle_model/vehicle_model/cal_roll_resi  Myu_tire=myu  Vehicle_Mass=M  Gravi_acc=g
  F_rollresi : Outport
  wires:
  V_tgt/1 -> cal_roll_resi1/1
  cal_roll_resi1/1 -> F_rollresi/1

== system METI_Thermal_ver01_Jmaab_2018b/Vehicle/ALT_PNT/Subsystem/I_alt_cal ==
  target_volt_ALT_V : Inport
  volt_BT_PNT_Lo_V : Inport  Port=2
  rpm_alt : Inport  Port=3
  Add : Sum
  Cal_I_alt_P_control : Subsystem
  Cal_I_alt_base : Subsystem
  Constant : Constant  Value=12
  Constant4 : Constant  Value=0
  Limit_Current_Max : Lookup_n-D  NumberOfTableDimensions=1  BreakpointsForDimension1=ALT_PNT_Alter_limit_Current_V_table_x_rpm  Table=ALT_PNT_Alter_limit_Current_V_table  ExtrapMethod=Clip  UseLastTableValue=on  RndMeth=Simplest  InputSameDT=on
  MinMax2 : MinMax  Function=max  Inputs=2
  Sum1 : Sum  Inputs=|+-
  Sum2 : Sum  Inputs=-+|
  電圧比較 : MinMax  Inputs=2
  I_alt : Outport
  wires:
  target_volt_ALT_V/1 -> Sum1/1, Sum2/2
  volt_BT_PNT_Lo_V/1 -> Sum2/1
  rpm_alt/1 -> Limit_Current_Max/1
  Constant4/1 -> MinMax2/2
  Limit_Current_Max/1 -> MinMax2/1  "I_limit_ALT"
  電圧比較/1 -> I_alt/1
  Add/1 -> 電圧比較/2
  Sum2/1 -> Cal_I_alt_P_control/1(V_delt_tgt)
  MinMax2/1 -> 電圧比較/1
  Constant/1 -> Sum1/2
  Sum1/1 -> Cal_I_alt_base/1(V_delt_tgt)
  Cal_I_alt_P_control/1(I_alt_base) -> Add/1
  Cal_I_alt_base/1(I_alt_base) -> Add/2

== system METI_Thermal_ver01_Jmaab_2018b/Vehicle/ALT_PNT/Subsystem/Torque_Guard ==
  current_ALT_PNT_A : Inport
  V_ALT_PNT : Inport  Port=2
  n_ROT_slavepulley12_rpm : Inport  Port=3
  ALT_GDCurrent : Inport  Port=4
  ALT_GDVolt : Inport  Port=5
  Caliculate_Axes_Torque1 : Lookup_n-D  NumberOfTableDimensions=3  BreakpointsForDimension1=ALT_PNT_Alter_trq_Nm_map_x_rpm  BreakpointsForDimension2=ALT_PNT_Alter_trq_Nm_map_y_Current_A  BreakpointsForDimension3=ALT_PNT_Alter_trq_Nm_map_z_Volt_tgt_V  Table=ALT_PNT_Alter_trq_Nm_map  RndMeth=Simplest  InputSameDT=on
  Caliculate_Axes_Torque2 : Lookup_n-D  NumberOfTableDimensions=3  BreakpointsForDimension1=ALT_PNT_Alter_trq_Nm_map_x_rpm  BreakpointsForDimension2=ALT_PNT_Alter_trq_Nm_map_y_Current_A  BreakpointsForDimension3=ALT_PNT_Alter_trq_Nm_map_z_Volt_tgt_V  Table=ALT_PNT_Alter_trq_Nm_map  RndMeth=Simplest  InputSameDT=on
  Constant3 : Constant  Value=ALT_PNT_trq_alter_output_LL_Nm
  MinMax : MinMax  Inputs=2
  MinMax1 : MinMax  Function=max  Inputs=2
  trq_trqsource : Outport
  wires:
  ALT_GDCurrent/1 -> Caliculate_Axes_Torque2/2
  Caliculate_Axes_Torque2/1 -> MinMax/2
  MinMax/1 -> MinMax1/1
  Caliculate_Axes_Torque1/1 -> MinMax/1
  Constant3/1 -> MinMax1/2
  ALT_GDVolt/1 -> Caliculate_Axes_Torque2/3
  MinMax1/1 -> trq_trqsource/1
  V_ALT_PNT/1 -> Caliculate_Axes_Torque1/3
  current_ALT_PNT_A/1 -> Caliculate_Axes_Torque1/2
  n_ROT_slavepulley12_rpm/1 -> Caliculate_Axes_Torque2/1, Caliculate_Axes_Torque1/1

== system METI_Thermal_ver01_Jmaab_2018b/Vehicle/BT_PNT_Lo/Cal_SOC/Subsystem4 ==
  In1 : Inport
  In2 : Inport  Port=2
  To Workspace : ToWorkspace  VariableName=SOC_LoBat  SampleTime=-1
      settings: Decimation=num_tws_mabiki
  To Workspace1 : ToWorkspace  VariableName=Asec_LoBat  SampleTime=-1
      settings: Decimation=num_tws_mabiki
  wires:
  In1/1 -> To Workspace/1
  In2/1 -> To Workspace1/1

== system METI_Thermal_ver01_Jmaab_2018b/Vehicle/CNT/ALT_CNT/ALT_Ctrl ==
  note: 【発電禁止条件】
      | 下記条件いずれかが成立時はオルタネータの発電を禁止する
      |   (2)エンジン停止中
      |   (3)エンジン始動中(下記エンジン回転数で判定)
      |      ene ≦ ALT_ON_RPM_HYS(1000[rpm])
      |                    ヒスあり(400[rpm])
  note: 【強制回生モード切替条件】
  note: 【回生モード切替条件】
      | 減速時FC中
  note: 例) 12[V]
  note: 例) 14[V]
  note: 例) 13.5[V]
  SOC_BT_PNT_Lo_PCT : Inport
  flag_fuelcut : Inport  Port=2
  flag_IdleStop : Inport  Port=3
  n_eng_rpm : Inport  Port=4
  Constant : Constant  Value=ALT_CNT_Alter_V_Kaisei_V
  Constant1 : Constant  Value=ALT_CNT_V_Battely_Kudo_V
  Constant2 : Constant  Value=ALT_CNT_flag_disable_kaisei
  Constant3 : Constant  Value=ALT_CNT_Alter_V_BASE_V
  Constant4 : Constant  Value=BT_PNT_Lo_SOC_MAX_lo_batt
  Logical Operator : Logic  Operator=OR  Inputs=3  AllPortsSameDT=off  OutDataTypeStr=boolean
  Logical Operator1 : Logic  AllPortsSameDT=off  OutDataTypeStr=boolean
  Logical Operator2 : Logic  Operator=NOT  AllPortsSameDT=off  OutDataTypeStr=boolean
  Relational Operator : RelationalOperator  OutDataTypeStr=boolean  RndMeth=Nearest
  Relay1 : Relay  OnSwitchValue=ALT_CNT_ALT_ON_RPM_HYS_rpm  OffSwitchValue=ALT_CNT_ALT_OFF_RPM_HYS_rpm  OnOutputValue=0  OffOutputValue=1
  Switch1 : Switch  Criteria=u2 > Threshold  Threshold=0.5
  Switch3 : Switch  Criteria=u2 > Threshold  Threshold=0.5
  target_volt_ALT_V : Outport
  wires:
  Switch3/1 -> target_volt_ALT_V/1  "target_volt_ALT_V"
  Constant3/1 -> Switch3/1
  Logical Operator2/1 -> Logical Operator1/2
  SOC_BT_PNT_Lo_PCT/1 -> Relational Operator/1
  Constant2/1 -> Switch3/2
  flag_fuelcut/1 -> Logical Operator1/1
  Relational Operator/1 -> Logical Operator/3
  Constant4/1 -> Relational Operator/2
  Logical Operator1/1 -> Switch1/2
  Logical Operator/1 -> Logical Operator2/1
  Constant/1 -> Switch1/1
  Relay1/1 -> Logical Operator/2
  Switch1/1 -> Switch3/3
  Constant1/1 -> Switch1/3
  flag_IdleStop/1 -> Logical Operator/1
  n_eng_rpm/1 -> Relay1/1

== system METI_Thermal_ver01_Jmaab_2018b/Vehicle/CNT/BK_CNT/BK_Ctrl ==
  open_brake_per_in : Inport
  open_brake_per : Outport
  wires:
  open_brake_per_in/1 -> open_brake_per/1

== system METI_Thermal_ver01_Jmaab_2018b/Vehicle/CNT/CAN/ALT_CNT ==
  note: ALT_Ctrl
  Pwtr_CAN : Inport
  Bus Creator2 : BusCreator  Inputs=3
  Bus Selector3 : BusSelector  OutputSignals=ENG_CNT_CAN_Tx
  Bus Selector4 : BusSelector  OutputSignals=flag_fuelcut,flag_IdleStop,n_eng_rpm
  tag scope: ALT_CNT_CAN_Rx=scoped
  wires:
  Bus Selector4/2 -> Bus Creator2/2  "<flag_IdleStop>"
  Bus Selector4/3 -> Bus Creator2/3  "<n_eng_rpm>"
  Pwtr_CAN/1 -> Bus Selector3/1
  Bus Creator2/1 -> [ALT_CNT_CAN_Rx]  "ALT_CNT_CAN_Rx"
  Bus Selector4/1 -> Bus Creator2/1  "<flag_fuelcut>"
  Bus Selector3/1 -> Bus Selector4/1  "<ENG_CNT_CAN_Tx>"

== system METI_Thermal_ver01_Jmaab_2018b/Vehicle/CNT/CAN/ENG_CNT ==
  note: ENG_Ctrl
  Pwtr_CAN : Inport
  Bus Creator3 : BusCreator  Inputs=1
  Bus Selector1 : BusSelector  OutputSignals=TM_CNT_CAN_Tx
  Bus Selector2 : BusSelector  OutputSignals=flag_Lockup
  ENG_CNT_CAN_Tx : Outport
  tag scope: ENG_CNT_CAN_Rx=scoped
  wires:
  Bus Creator3/1 -> [ENG_CNT_CAN_Rx]  "ENG_CNT_CAN_Rx"
  Bus Selector1/1 -> Bus Selector2/1  "<TM_CNT_CAN_Tx>"
  Bus Selector2/1 -> Bus Creator3/1  "<flag_Lockup>"
  Pwtr_CAN/1 -> Bus Selector1/1
  [ENG_CNT_CAN_Tx] -> ENG_CNT_CAN_Tx/1

== system METI_Thermal_ver01_Jmaab_2018b/Vehicle/CNT/CAN/Pwtr_CAN ==
  note: 通信遅れ無し
  ENG_CNT_CAN_Tx : Inport
  TM_CNT_CAN_Tx : Inport  Port=2
  Bus Creator8 : BusCreator  Inputs=2
  Pwtr_CAN : Outport
  wires:
  ENG_CNT_CAN_Tx/1 -> Bus Creator8/1
  TM_CNT_CAN_Tx/1 -> Bus Creator8/2
  Bus Creator8/1 -> Pwtr_CAN/1  "Pwtr_CAN"

== system METI_Thermal_ver01_Jmaab_2018b/Vehicle/CNT/CAN/TM_CNT ==
  note: TM_Ctrl
  Pwtr_CAN : Inport
  Bus Creator4 : BusCreator  Inputs=1
  Bus Selector5 : BusSelector  OutputSignals=ENG_CNT_CAN_Tx
  Bus Selector6 : BusSelector  OutputSignals=open_throttle_per
  TM_CNT_CAN_Tx : Outport
  tag scope: TM_CNT_CAN_Rx=scoped
  wires:
  Bus Selector5/1 -> Bus Selector6/1  "<ENG_CNT_CAN_Tx>"
  Bus Selector6/1 -> Bus Creator4/1  "<open_throttle_per>"
  Pwtr_CAN/1 -> Bus Selector5/1
  Bus Creator4/1 -> [TM_CNT_CAN_Rx]  "TM_CNT_CAN_Rx"
  [TM_CNT_CAN_Tx] -> TM_CNT_CAN_Tx/1

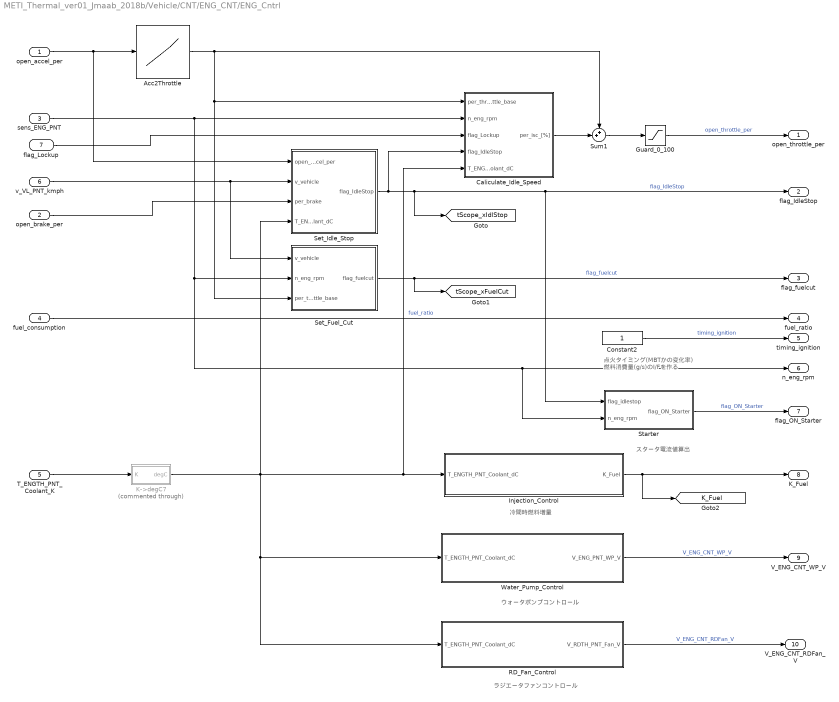
== system METI_Thermal_ver01_Jmaab_2018b/Vehicle/CNT/ENG_CNT/ENG_Cntrl ==
  note: 点火タイミング(MBTかの変化率)
      | 燃料消費量(g/s)のI/Fを作る
  note: スタータ電流値算出
  note: 冷間時燃料増量
  note: ウォータポンプコントロール
  note: ラジエータファンコントロール
  open_accel_per : Inport
  open_brake_per : Inport  Port=2
  sens_ENG_PNT : Inport  Port=3
  fuel_consumption : Inport  Port=4
  T_ENGTH_PNT_Coolant_K : Inport  Port=5
  v_VL_PNT_kmph : Inport  Port=6
  flag_Lockup : Inport  Port=7
  Acc2Throttle : Lookup_n-D  NumberOfTableDimensions=1  BreakpointsForDimension1=[ENG_CNT_Accel_LL:ENG_CNT_Accel_UL]  Table=[ENG_CNT_Throttle_LL:ENG_CNT_Throttle_UL]  RndMeth=Simplest  InputSameDT=on
  Caliculate_Idle_Speed : Subsystem
  Constant2 : Constant
  Guard_0_100 : Saturate  UpperLimit=ENG_CNT_Throttle_UL  LowerLimit=ENG_CNT_Throttle_LL
  Injection_Control : Subsystem
  K->degC7 : Subsystem  Commented=through
  RD_Fan_Control : Subsystem
  Set_Fuel_Cut : Subsystem
  Set_Idle_Stop : Subsystem
  Starter : Subsystem
  Sum1 : Sum  Inputs=++|
  Water_Pump_Control : Subsystem
  open_throttle_per : Outport
  flag_IdleStop : Outport  Port=2
  flag_fuelcut : Outport  Port=3
  fuel_ratio : Outport  Port=4
  timing_ignition : Outport  Port=5
  n_eng_rpm : Outport  Port=6
  flag_ON_Starter : Outport  Port=7
  K_Fuel : Outport  Port=8
  V_ENG_CNT_WP_V : Outport  Port=9
  V_ENG_CNT_RDFan_V : Outport  Port=10
  tag scope: K_Fuel=global, tScope_xFuelCut=global, tScope_xIdlStop=global
  wires:
  Set_Idle_Stop/1(flag_IdleStop) -> [tScope_xIdlStop], Starter/1(flag_idlestop), flag_IdleStop/1, Caliculate_Idle_Speed/4(flag_IdleStop)  "flag_IdleStop"
  Caliculate_Idle_Speed/1(per_isc_[%]) -> Sum1/2
  Sum1/1 -> Guard_0_100/1
  Acc2Throttle/1 -> Sum1/1, Caliculate_Idle_Speed/1(per_throttle_base), Set_Fuel_Cut/3(per_throttle_base)
  fuel_consumption/1 -> fuel_ratio/1  "fuel_ratio"
  Constant2/1 -> timing_ignition/1  "timing_ignition"
  Set_Fuel_Cut/1(flag_fuelcut) -> flag_fuelcut/1, [tScope_xFuelCut]  "flag_fuelcut"
  Guard_0_100/1 -> open_throttle_per/1  "open_throttle_per"
  sens_ENG_PNT/1 -> Caliculate_Idle_Speed/2(n_eng_rpm), Set_Fuel_Cut/2(n_eng_rpm), n_eng_rpm/1, Starter/2(n_eng_rpm)
  open_brake_per/1 -> Set_Idle_Stop/3(per_brake)
  open_accel_per/1 -> Acc2Throttle/1, Set_Idle_Stop/1(open_accel_per)
  v_VL_PNT_kmph/1 -> Set_Fuel_Cut/1(v_vehicle), Set_Idle_Stop/2(v_vehicle)
  Starter/1(flag_ON_Starter) -> flag_ON_Starter/1  "flag_ON_Starter"
  flag_Lockup/1 -> Caliculate_Idle_Speed/3(flag_Lockup)
  Water_Pump_Control/1(V_ENG_PNT_WP_V) -> V_ENG_CNT_WP_V/1  "V_ENG_CNT_WP_V"
  T_ENGTH_PNT_Coolant_K/1 -> K->degC7/1(K)
  Injection_Control/1(K_Fuel) -> [K_Fuel], K_Fuel/1
  RD_Fan_Control/1(V_RDTH_PNT_Fan_V) -> V_ENG_CNT_RDFan_V/1  "V_ENG_CNT_RDFan_V"
  K->degC7/1(degC) -> RD_Fan_Control/1(T_ENGTH_PNT_Coolant_dC), Water_Pump_Control/1(T_ENGTH_PNT_Coolant_dC), Set_Idle_Stop/4(T_ENGTH_PNT_Coolant_dC), Injection_Control/1(T_ENGTH_PNT_Coolant_dC), Caliculate_Idle_Speed/5(T_ENGTH_PNT_Coolant_dC)

== system METI_Thermal_ver01_Jmaab_2018b/Vehicle/CNT/TM_CNT/TM_Ctrl ==
  v_VL_PNT_kmph : Inport
  n_TM_PNT_rpm : Inport  Port=2
  T_TMTH_PNT_CVTF_K : Inport  Port=3
  T_ENG_Coolant_K : Inport  Port=4
  open_throttle_per : Inport  Port=5
  CVT_ECU : Subsystem
  K->degC : Subsystem  Commented=through
  K->degC1 : Subsystem  Commented=through
  LockupClutch_ECU : Subsystem
  Memory{,1..4} (5 alike) : Memory
  WarmerECU : Subsystem
  flag_Lockup : Outport
  omg_Slip_rpm : Outport  Port=2
  ratio_CVT : Outport  Port=3
  R_CVTF_warmer_tgt_KpW : Outport  Port=4
  tag scope: tScope_CVTratio=global, tScope_Luckup=global
  wires:
  CVT_ECU/1(ratio_CVT) -> [tScope_CVTratio], ratio_CVT/1  "ratio_CVT"
  LockupClutch_ECU/1(flag_Lockup) -> [tScope_Luckup], flag_Lockup/1  "flag_Lockup"
  LockupClutch_ECU/2(omg_Slip_rpm) -> omg_Slip_rpm/1  "omg_Slip_rpm"
  open_throttle_per/1 -> Memory1/1
  Memory/1 -> LockupClutch_ECU/1(v_vehicle)
  Memory1/1 -> CVT_ECU/1(per_throttle), LockupClutch_ECU/2(per_throttle)
  Memory2/1 -> CVT_ECU/2(omg_pera)
  n_TM_PNT_rpm/1 -> Memory2/1
  v_VL_PNT_kmph/1 -> Memory/1
  T_TMTH_PNT_CVTF_K/1 -> Memory3/1
  T_ENG_Coolant_K/1 -> Memory4/1
  Memory3/1 -> K->degC/1(K)
  Memory4/1 -> K->degC1/1(K)
  WarmerECU/1(R_CVTF_warmer_tgt_KpW) -> R_CVTF_warmer_tgt_KpW/1  "R_CVTF_warmer_tgt_KpW"
  K->degC/1(degC) -> WarmerECU/1(T_TMTH_PNT_CVTF_dC)
  K->degC1/1(degC) -> WarmerECU/2(T_ENG_Coolant_dC)

== system METI_Thermal_ver01_Jmaab_2018b/Vehicle/ENG_PNT/ENG_Plant/Cal_FuelComsunption ==
  w_ENG_PNT_radps : Inport
  trq_ENG : Inport  Port=2
  flag_fuelcut : Inport  Port=3
  flag_IdleStop : Inport  Port=4
  timing_ignition : Inport  Port=5
  K_Fuel : Inport  Port=6
  1-D Lookup Table1 : Lookup_n-D  NumberOfTableDimensions=1  BreakpointsForDimension1=ENG_PNT_trq_fluc_Nm_table_x_spk_tim  Table=ENG_PNT_trq_fluc_Nm_table  RndMeth=Simplest  InputSameDT=on
  Map_FuelRate : Lookup_n-D  BreakpointsForDimension1=ENG_PNT_FuelCon_gps_map_y_trq_Nm  BreakpointsForDimension2=ENG_PNT_FuelCon_gps_map_x_pri_rpm  Table=ENG_PNT_FuelCon_gps_map  RndMeth=Simplest  InputSameDT=on
  Not_cal1 : Subsystem
  Not_cal2 : Subsystem
  Product : Product  Inputs=4  RndMeth=Zero
  Product1 : Product  Inputs=*/  RndMeth=Zero
  radpsec2rpm : Gain  Gain=radpsec2rpm
  FuelConsumption : Outport
  wires:
  trq_ENG/1 -> Product1/1
  radpsec2rpm/1 -> Map_FuelRate/2
  w_ENG_PNT_radps/1 -> radpsec2rpm/1
  Product/1 -> FuelConsumption/1
  Not_cal2/1(Out1) -> Product/3
  Not_cal1/1(Out1) -> Product/2
  flag_fuelcut/1 -> Not_cal1/1(In1)
  flag_IdleStop/1 -> Not_cal2/1(In1)
  timing_ignition/1 -> 1-D Lookup Table1/1
  1-D Lookup Table1/1 -> Product1/2
  Product1/1 -> Map_FuelRate/1
  Map_FuelRate/1 -> Product/1
  K_Fuel/1 -> Product/4

== system METI_Thermal_ver01_Jmaab_2018b/Vehicle/ENG_PNT/ENG_Plant/Cal_trq_ENG_jiku ==
  note: エンジン軸トルクマップ
  open_throttle_per : Inport
  flag_fuelcut : Inport  Port=2
  flag_IdleStop : Inport  Port=3
  timing_ignition : Inport  Port=4
  w_ENG_PNT_radps : Inport  Port=5
  1-D Lookup Table : Lookup_n-D  NumberOfTableDimensions=1  BreakpointsForDimension1=ENG_PNT_trq_fluc_Nm_table_x_spk_tim  Table=ENG_PNT_trq_fluc_Nm_table  RndMeth=Simplest  InputSameDT=on
  2-D Lookup Table : Lookup_n-D  BreakpointsForDimension1=ENG_PNT_trq_Nm_map_y_throttle  BreakpointsForDimension2=ENG_PNT_trq_Nm_map_x_rpm  Table=ENG_PNT_trq_Nm_map  ExtrapMethod=Clip  UseLastTableValue=on  RndMeth=Simplest  InputSameDT=on
  Model Info : simulink/Model-Wide Utilities/Model Info  Frame=on  DisplayStringWithTags=|  HorizontalTextAlignment=Left  LeftAlignmentValue=0.02
      | 【注記】
      | ・燃料カット時はスロットル開度を0としてエンジンフリクションを付加
      | ・点火タイミングによるトルク変動を想定
      | ・エンジン軸トルクマップの使用
  Not_cal : Subsystem
  Not_cal1 : Subsystem
  Product : Product  RndMeth=Zero
  Product1 : Product  RndMeth=Zero
  Product2 : Product  RndMeth=Zero
  Saturation : Saturate  UpperLimit=ENG_CNT_Throttle_UL  LowerLimit=ENG_CNT_Throttle_LL
  radpsec2rpm : Gain  Gain=radpsec2rpm
  trq_ENG_PNT_Nm : Outport
  wires:
  w_ENG_PNT_radps/1 -> radpsec2rpm/1
  2-D Lookup Table/1 -> Product1/1
  open_throttle_per/1 -> Product/1
  Saturation/1 -> 2-D Lookup Table/1
  radpsec2rpm/1 -> 2-D Lookup Table/2
  timing_ignition/1 -> 1-D Lookup Table/1
  1-D Lookup Table/1 -> Product1/2
  Product/1 -> Saturation/1
  Product2/1 -> Product/2
  flag_fuelcut/1 -> Not_cal/1(In1)
  Not_cal/1(Out1) -> Product2/1
  flag_IdleStop/1 -> Not_cal1/1(In1)
  Not_cal1/1(Out1) -> Product2/2
  Product1/1 -> trq_ENG_PNT_Nm/1  "trq_ENG_PNT_Nm"

== system METI_Thermal_ver01_Jmaab_2018b/Vehicle/ENG_PNT/ENG_Plant/Coldstart_Additional_friction_calc2 ==
  note: スロットル開度0の時の
      | 軸トルクを読み出し
  T_ENGOil_degC : Inport
  w_ENG_PNT_radps : Inport  Port=2
  1-D Lookup Table : Lookup_n-D  NumberOfTableDimensions=1  BreakpointsForDimension1=ENG_PNT_Cold_friction_gain_x_T_ENGOil  Table=ENG_PNT_Cold_friction_gain  InternalRulePriority=Speed  RndMeth=Simplest  InputSameDT=on
  2-D Lookup Table : Lookup_n-D  BreakpointsForDimension1=ENG_PNT_trq_Nm_map_y_throttle  BreakpointsForDimension2=ENG_PNT_trq_Nm_map_x_rpm  Table=ENG_PNT_trq_Nm_map  ExtrapMethod=Clip  UseLastTableValue=on  RndMeth=Simplest  InputSameDT=on
  Add : Sum  Inputs=+-
  Constant1 : Constant  Value=0
  Product : Product
  radpsec2rpm : Gain  Gain=radpsec2rpm
  Additional_friction : Outport
  wires:
  T_ENGOil_degC/1 -> 1-D Lookup Table/1
  w_ENG_PNT_radps/1 -> radpsec2rpm/1
  radpsec2rpm/1 -> 2-D Lookup Table/2
  Constant1/1 -> 2-D Lookup Table/1
  2-D Lookup Table/1 -> Add/2, Product/2
  1-D Lookup Table/1 -> Product/1
  Add/1 -> Additional_friction/1
  Product/1 -> Add/1

== system METI_Thermal_ver01_Jmaab_2018b/Vehicle/ENG_PNT/ENG_Plant/Coldstart_Heat_flux_gain_calc ==
  T_ENGOil_degC : Inport
  1-D Lookup Table : Lookup_n-D  NumberOfTableDimensions=1  BreakpointsForDimension1=ENG_PNT_Heatflux2ENGOil_gain_x_T_ENGOil  Table=ENG_PNT_Heatflux2ENGOil_gain  InternalRulePriority=Speed  RndMeth=Simplest  InputSameDT=on
  Heat_flux_gain : Outport
  wires:
  T_ENGOil_degC/1 -> 1-D Lookup Table/1
  1-D Lookup Table/1 -> Heat_flux_gain/1

== system METI_Thermal_ver01_Jmaab_2018b/Vehicle/ENG_PNT/ENG_Plant/Coldstart_Heat_flux_gain_calc1 ==
  T_ENG_Cylinder_Head_degC : Inport
  1-D Lookup Table : Lookup_n-D  NumberOfTableDimensions=1  BreakpointsForDimension1=ENG_PNT_Heatflux2Cylinder_Head_gain_x_T_Coolant  Table=ENG_PNT_Heatflux2Cylinder_Head_gain  InternalRulePriority=Speed  RndMeth=Simplest  InputSameDT=on
  Heat_flux_gain : Outport
  wires:
  T_ENG_Cylinder_Head_degC/1 -> 1-D Lookup Table/1
  1-D Lookup Table/1 -> Heat_flux_gain/1

== system METI_Thermal_ver01_Jmaab_2018b/Vehicle/ENG_PNT/ENG_Plant/K->degC1 ==
  K : Inport
  Constant2 : Constant  Value=K2degC
  Sum : Sum  Inputs=++|
  degC : Outport
  wires:
  K/1 -> Sum/2
  Constant2/1 -> Sum/1
  Sum/1 -> degC/1

== system METI_Thermal_ver01_Jmaab_2018b/Vehicle/ENG_PNT/ENG_Plant/K->degC6 ==
  K : Inport
  Constant2 : Constant  Value=K2degC
  Sum : Sum  Inputs=++|
  degC : Outport
  wires:
  K/1 -> Sum/2
  Constant2/1 -> Sum/1
  Sum/1 -> degC/1

== system METI_Thermal_ver01_Jmaab_2018b/Vehicle/PTTH/ATM_PNT/degC->K ==
  degC : Inport
  Constant2 : Constant  Value=degC2K
  Sum : Sum  Inputs=++|
  K : Outport
  wires:
  degC/1 -> Sum/2
  Constant2/1 -> Sum/1
  Sum/1 -> K/1

== system METI_Thermal_ver01_Jmaab_2018b/Vehicle/PTTH/ATM_PNT/degC->K1 ==
  degC : Inport
  Constant2 : Constant  Value=degC2K
  Sum : Sum  Inputs=++|
  K : Outport
  wires:
  Sum/1 -> K/1
  Constant2/1 -> Sum/1
  degC/1 -> Sum/2

== system METI_Thermal_ver01_Jmaab_2018b/Vehicle/PTTH/ATM_PNT/degC->K2 ==
  degC : Inport
  Constant2 : Constant  Value=degC2K
  Sum : Sum  Inputs=++|
  K : Outport
  wires:
  degC/1 -> Sum/2
  Constant2/1 -> Sum/1
  Sum/1 -> K/1

== system METI_Thermal_ver01_Jmaab_2018b/Vehicle/PTTH/ATM_PNT/degC->K3 ==
  degC : Inport
  Constant2 : Constant  Value=degC2K
  Sum : Sum  Inputs=++|
  K : Outport
  wires:
  Sum/1 -> K/1
  Constant2/1 -> Sum/1
  degC/1 -> Sum/2

== system METI_Thermal_ver01_Jmaab_2018b/Vehicle/PTTH/DTTH_PNT/DFTH_PNT ==
  note: T/Mブロックから
      | 受け取る熱量
  note: DFオイルの
      | 熱容量
  note: DFブロックの
      | 熱容量
  note: DFの損失が
      | DFオイルへの熱量
  note: エネルギーの
      | 向きの定義（仮）
      | →→→
  note: エネルギーの
      | 向きの定義（仮）
      | →→→
  note: エネルギーの
      | 向きの定義（仮）
      | →→→
  note: エネルギーの
      | 向きの定義（仮）
      | →→→
  note: エネルギーの
      | 向きの定義（仮）
      | →→→
  T_DF_Block_K : Inport
  PHI_DF_PNT_W : Inport  Port=2
  T_ATM_PNT_DF_K : Inport  Port=3
  DFBlock_Heat_Capacity : Subsystem
  DFOil2DFBlock_Heat_Resistance : Subsystem
  DFOil_Heat_Capacity : Subsystem
  ENGBlock2Air_Heat_Resistance : Subsystem
  TMBlock2DFBlock_Heat_Resistance : Subsystem
  Terminator : Terminator
  PHI_DF_Block_W : Outport
  PHI_DFTH_PNT_W : Outport  Port=2
  T_DFBlock_K : Outport  Port=3
  wires:
  DFOil_Heat_Capacity/1(T_DFOil2_K) -> DFOil2DFBlock_Heat_Resistance/1(T_DFOil_Resi2_K)
  DFOil2DFBlock_Heat_Resistance/1(PHI_DFOil_Resi2_W) -> DFOil_Heat_Capacity/1(PHI_DFOil2_W)
  DFBlock_Heat_Capacity/3(T_DFBlock1_K) -> DFOil2DFBlock_Heat_Resistance/2(T_DFBlock_Resi_K)
  DFOil2DFBlock_Heat_Resistance/2(PHI_DFBlock_Resi_W) -> DFBlock_Heat_Capacity/3(PHI_DFBlock1_W)
  ENGBlock2Air_Heat_Resistance/1(PHI_DFBlock_Resi_W) -> DFBlock_Heat_Capacity/1(PHI_DFBlock3_W)
  DFBlock_Heat_Capacity/2(T_DFBlock3_K) -> ENGBlock2Air_Heat_Resistance/1(T_DFBlock_Resi_K)
  T_ATM_PNT_DF_K/1 -> ENGBlock2Air_Heat_Resistance/2(T_DF_Air_Resi_K)
  ENGBlock2Air_Heat_Resistance/2(PHI_DF_Air_Resi_W) -> PHI_DFTH_PNT_W/1  "PHI_DFTH_PNT_W"
  T_DF_Block_K/1 -> TMBlock2DFBlock_Heat_Resistance/2(T_TMBlock_Resi_K)
  TMBlock2DFBlock_Heat_Resistance/2(PHI_TMBlock_Resi_W) -> PHI_DF_Block_W/1  "PHI_DF_Block_W"
  TMBlock2DFBlock_Heat_Resistance/1(PHI_DFBlock_Resi_W) -> DFBlock_Heat_Capacity/2(PHI_DFBlock2_W)
  DFBlock_Heat_Capacity/1(T_DFBlock2_K) -> T_DFBlock_K/1, TMBlock2DFBlock_Heat_Resistance/1(T_DFBlock_Resi_K)  "T_DFBlock_K"
  DFOil_Heat_Capacity/2(T_DFOil1_K) -> Terminator/1
  PHI_DF_PNT_W/1 -> DFOil_Heat_Capacity/2(PHI_DFOil1_W)

== system METI_Thermal_ver01_Jmaab_2018b/Vehicle/PTTH/DTTH_PNT/TMTH_PNT ==
  note: CVTFの
      | 熱容量
  note: T/Mブロックの
      | 熱容量
  note: DFブロックへ
      | 放熱する熱量
  note: エンジンブロックから
      | 受け取る熱量
  note: CVTFからエンジン冷却水へ
      | 放熱する熱量
  note: T/Mの入力-出力が
      | CVTFへの熱量
  note: エネルギーの
      | 向きの定義（仮）
      | ←←←
  note: エネルギーの
      | 向きの定義（仮）
      | →→→
  note: エネルギーの
      | 向きの定義（仮）
      | →→→
  note: エネルギーの
      | 向きの定義（仮）
      | →→→
  note: エネルギーの
      | 向きの定義（仮）
      | →→→
  note: エネルギーの
      | 向きの定義（仮）
      | →→→
  note: エネルギーの
      | 向きの定義（仮）
      | →→→
  note: TMブロックからから大気へ
      | 放熱する熱量
  W_TM_Block0_W : Inport
  R_CVTF_warmer_tgt_KpW : Inport  Port=2
  PHI_TM_PNT_W : Inport  Port=3
  T_TM_Block_Resi_K : Inport  Port=4
  T_ENGTH_PNT_Coolant_K : Inport  Port=5
  T_ATM_PNT_TM_K : Inport  Port=6
  CVTF2Coolant_Heat_Resistance : Subsystem
  CVTF2TMBlock_Heat_Resistance : Subsystem
  CVTF_Heat_Capacity : Subsystem
  ENGBlock2TMBlock_Heat_Resistance : Subsystem
  TMBlock2Air_Heat_Resistance : Subsystem
  TMBlock_Heat_Capacity : Subsystem
  T_TMTH_PNT_CVTF1_K : Outport
  T_TM_Block0_K : Outport  Port=2
  PHI_TM_CVTF_Resi_W : Outport  Port=3
  T_TMTH_PNT_CVTF_K : Outport  Port=4
  PHI_ENGBlock_Resi2_W : Outport  Port=5
  PHI_TMTH_PNT_W : Outport  Port=6
  tag scope: R_CVTF_warmer_tgt_KpW=global
  wires:
  CVTF_Heat_Capacity/1(T_CVTF4_K) -> CVTF2TMBlock_Heat_Resistance/1(T_CVTF_Resi4_K)
  CVTF2TMBlock_Heat_Resistance/1(PHI_CVTF_Resi4_W) -> CVTF_Heat_Capacity/1(PHI_CVTF4_W)
  TMBlock_Heat_Capacity/4(T_TMBlock1_K) -> CVTF2TMBlock_Heat_Resistance/2(T_TMBlock_Resi1_K)
  CVTF2TMBlock_Heat_Resistance/2(PHI_TMBlock_Resi1_W) -> TMBlock_Heat_Capacity/3(PHI_TMBlock1_W)
  CVTF_Heat_Capacity/3(T_CVTF1_K) -> T_TMTH_PNT_CVTF_K/1, T_TMTH_PNT_CVTF1_K/1  "T_TMTH_PNT_CVTF_K"
  PHI_TM_PNT_W/1 -> CVTF_Heat_Capacity/2(PHI_CVTF1_W)
  TMBlock2Air_Heat_Resistance/1(PHI_TMBlock_Resi3_W) -> TMBlock_Heat_Capacity/1(PHI_TMBlock3_W)
  TMBlock_Heat_Capacity/2(T_TMBlock3_K) -> TMBlock2Air_Heat_Resistance/1(T_TMBlock_Resi3_K)
  T_ATM_PNT_TM_K/1 -> TMBlock2Air_Heat_Resistance/2(T_TM_Air_Resi1_K)
  TMBlock2Air_Heat_Resistance/2(PHI_TM_Air_Resi1_W) -> PHI_TMTH_PNT_W/1  "PHI_TMTH_PNT_W"
  T_TM_Block_Resi_K/1 -> ENGBlock2TMBlock_Heat_Resistance/2(T_ENGBlock_Resi2_K)
  ENGBlock2TMBlock_Heat_Resistance/2(PHI_ENGBlock_Resi2_W) -> PHI_ENGBlock_Resi2_W/1  "PHI_ENGBlock_Resi2_W"
  CVTF_Heat_Capacity/2(T_CVTF2_K) -> CVTF2Coolant_Heat_Resistance/1(T_CVTF_Resi2_K)
  CVTF2Coolant_Heat_Resistance/2(PHI_CVTF_Resi2_W) -> CVTF_Heat_Capacity/3(PHI_CVT2_W)
  CVTF2Coolant_Heat_Resistance/1(PHI_Coolant_Resi2_W) -> PHI_TM_CVTF_Resi_W/1  "PHI_TM_CVTF_Resi_W"
  T_ENGTH_PNT_Coolant_K/1 -> CVTF2Coolant_Heat_Resistance/3(T_Coolant_Resi2_K)
  ENGBlock2TMBlock_Heat_Resistance/1(PHI_TMBlock_Resi2_W) -> TMBlock_Heat_Capacity/2(PHI_TMBlock2_W)
  TMBlock_Heat_Capacity/1(T_TMBlock2_K) -> ENGBlock2TMBlock_Heat_Resistance/1(T_TMBlock_Resi2_K)
  TMBlock_Heat_Capacity/3(T_TMBlock4_K) -> T_TM_Block0_K/1  "T_TM_Block0_degC"
  W_TM_Block0_W/1 -> TMBlock_Heat_Capacity/4(PHI_TMBlock4_W)
  R_CVTF_warmer_tgt_KpW/1 -> CVTF2Coolant_Heat_Resistance/2(R_CVTF_warmer_tgt_KpW), [R_CVTF_warmer_tgt_KpW]
